simulink model "lab1"  (R2016a)
settings: Solver=VariableStepAuto  StartTime=0.0  StopTime=10.0  RelTol=1e-3
settings Model: Creator=ms36124  LastModifiedBy=ms36124

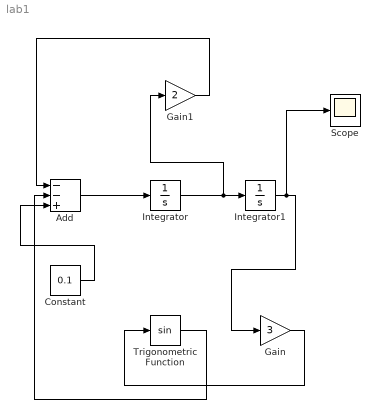
== system lab1 ==
  Add : Sum  Inputs=--+
  Constant : Constant  Value=0.1
  Gain : Gain  Gain=3
  Gain1 : Gain  Gain=2
  Integrator : Integrator  InitialCondition=2
  Integrator1 : Integrator
  Scope : Scope
  Trigonometric Function : Trigonometry
  wires:
  Add/1 -> Integrator/1
  Integrator/1 -> Gain1/1, Integrator1/1
  Gain1/1 -> Add/1
  Integrator1/1 -> Scope/1, Gain/1
  Gain/1 -> Trigonometric Function/1
  Trigonometric Function/1 -> Add/2
  Constant/1 -> Add/3
